simulink model "project_2023_11_27_p66_1"  (R2017b)
settings: Solver=VariableStepAuto  StartTime=0.0  StopTime=50  RelTol=1e-3
settings Model: Creator=Administrator  LastModifiedBy=Administrator

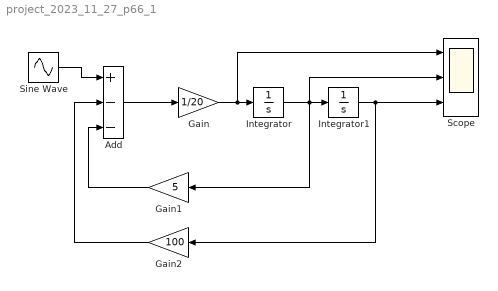
== system project_2023_11_27_p66_1 ==
  Add : Sum  Inputs=+--
  Gain : Gain  Gain=1/20
  Gain1 : Gain  Gain=5
  Gain2 : Gain  Gain=100
  Integrator : Integrator
  Integrator1 : Integrator
  Scope : Scope  NumInputPorts=3
  Sine Wave : Sin  Amplitude=4  Frequency=5  SampleTime=0
  wires:
  Add/1 -> Gain/1
  Gain/1 -> Scope/1, Integrator/1
  Integrator/1 -> Gain1/1, Scope/2, Integrator1/1
  Integrator1/1 -> Gain2/1, Scope/3
  Gain1/1 -> Add/3
  Gain2/1 -> Add/2
  Sine Wave/1 -> Add/1
